simulink model "ModelArticulatingSpacecraftSolarPanelsforSunTrackingExample"  (R2025b)
settings: Solver=ode45  StartTime=0.0  StopTime=endTime  FixedStep=1/60  MaxStep=10  RelTol=1e-10  AbsTol=1e-10
undefined symbols (not defined in the file or in its folder): juliandate, panelY
libraries: aerolibutil x10, simulink x6, simulink_extras x6, aerolibsatdyn x4
settings Model: Creator=The MathWorks, Inc.  LastModifiedBy=Trent Jerome
settings OptimizationCC: ReuseModelBlockBuffer=off
settings ModelReferenceCC: EnableRefExpFcnMdlSchedulingChecks=on
settings RTWCC: GPUComputeCapability=3.5

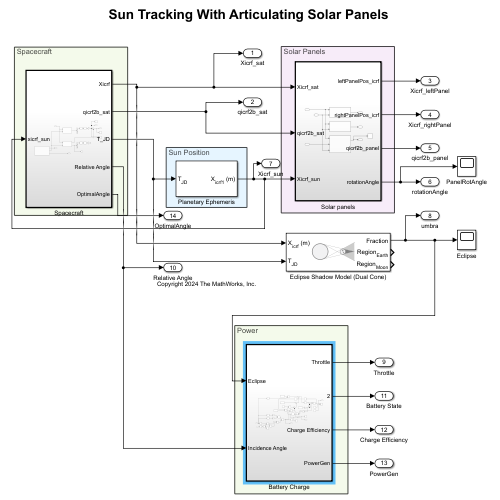
[thumbnail: Simulink's stored preview of the top-level diagram]
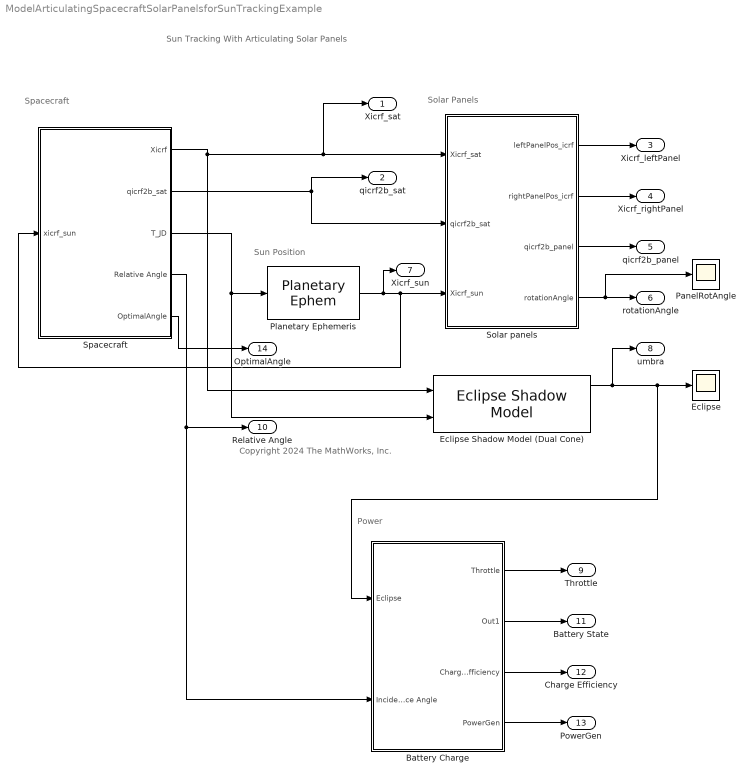
== system ModelArticulatingSpacecraftSolarPanelsforSunTrackingExample ==
  note: Sun Position
  note: Spacecraft
  note: Sun Tracking With Articulating Solar Panels
  note: Copyright 2024 The MathWorks, Inc.
  note: Solar Panels
  note: Power
  Battery Charge : Subsystem  TreatAsAtomicUnit=on
  Eclipse : Scope
      settings: ActiveDisplayYMinimum=-0.12499999999999997  ActiveDisplayYMaximum=1.125  DataLoggingVariableName=ScopeData2
  Eclipse Shadow Model (Dual Cone) : EclipseShadowModel  outputShadowRegion=on  timeSource=Port (Julian date)  useEphemerisDateRange=off  ephemerisEndDate=juliandate(2040, 1, 1)  action=Warning
  PanelRotAngle : Scope
      settings: ActiveDisplayYMinimum=0.6065745888777152  ActiveDisplayYMaximum=1.1603570435787431  DataLoggingVariableName=ScopeData12
  Planetary Ephemeris : PlanetaryEphem  units=m,m/s  target=Sun  outputVelocity=off
  Solar panels : Subsystem  TreatAsAtomicUnit=on
  Spacecraft : Subsystem  TreatAsAtomicUnit=on
  Xicrf_sat : Outport
  qicrf2b_sat : Outport  Port=2
  Xicrf_leftPanel : Outport  Port=3
  Xicrf_rightPanel : Outport  Port=4
  qicrf2b_panel : Outport  Port=5
  rotationAngle : Outport  Port=6
  Xicrf_sun : Outport  Port=7
  umbra : Outport  Port=8
  Throttle : Outport  Port=9
  Relative Angle : Outport  Port=10
  Battery State : Outport  Port=11
  Charge Efficiency : Outport  Port=12
  PowerGen : Outport  Port=13
  OptimalAngle : Outport  Port=14
  wires:
  Spacecraft/3(T_JD) -> Eclipse Shadow Model (Dual Cone)/2, Planetary Ephemeris/1
  Spacecraft/2(qicrf2b_sat) -> Solar panels/2(qicrf2b_sat), qicrf2b_sat/1
  Solar panels/2(rightPanelPos_icrf) -> Xicrf_rightPanel/1
  Solar panels/3(qicrf2b_panel) -> qicrf2b_panel/1
  Planetary Ephemeris/1 -> Xicrf_sun/1, Spacecraft/1(xicrf_sun), Solar panels/3(Xicrf_sun)
  Solar panels/1(leftPanelPos_icrf) -> Xicrf_leftPanel/1
  Solar panels/4(rotationAngle) -> PanelRotAngle/1, rotationAngle/1
  Spacecraft/1(Xicrf) -> Eclipse Shadow Model (Dual Cone)/1, Xicrf_sat/1, Solar panels/1(Xicrf_sat)
  Eclipse Shadow Model (Dual Cone)/1 -> umbra/1, Battery Charge/1(Eclipse), Eclipse/1
  Battery Charge/1(Throttle) -> Throttle/1
  Spacecraft/4(Relative Angle) -> Battery Charge/2(Incidence Angle), Relative Angle/1
  Battery Charge/2(Out1) -> Battery State/1
  Battery Charge/3(Charge Efficiency) -> Charge Efficiency/1
  Battery Charge/4(PowerGen) -> PowerGen/1
  Spacecraft/5(OptimalAngle) -> OptimalAngle/1

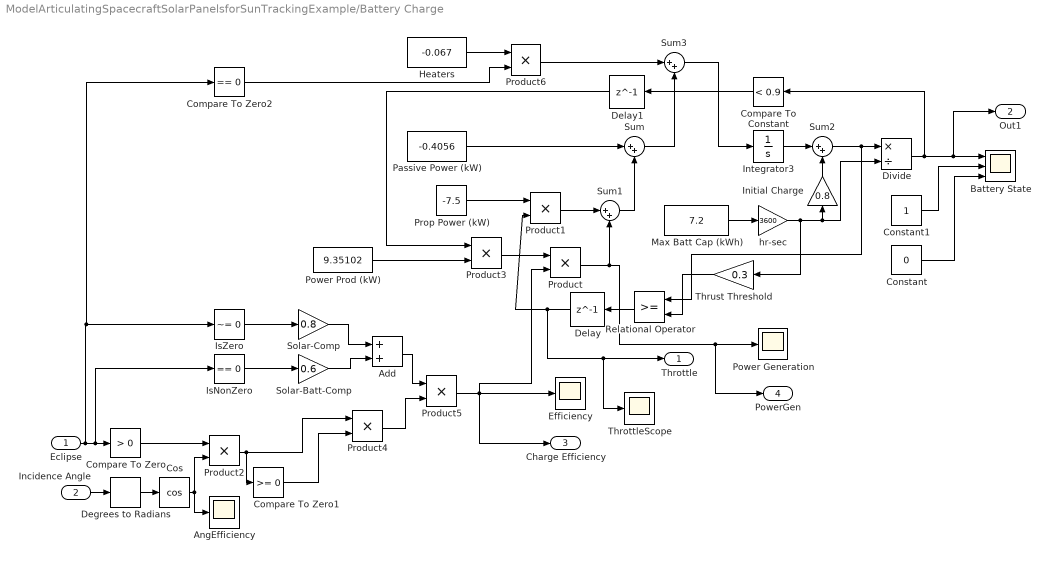
== system ModelArticulatingSpacecraftSolarPanelsforSunTrackingExample/Battery Charge ==
  Eclipse : Inport
  Incidence Angle : Inport  Port=2
  Add : Sum
  AngEfficiency : Scope
      settings: ActiveDisplayYMinimum=0.84489373386361877  ActiveDisplayYMaximum=1.0172340295545648  DataLoggingVariableName=ScopeData8
  Battery State : Scope  NumInputPorts=3
      settings: ActiveDisplayYMinimum=-0.12499999999999997  ActiveDisplayYMaximum=1.125  DataLoggingVariableName=ScopeData6
  Compare To Constant : simulink/Logic and Bit Operations/Compare To Constant  relop=<  const=0.9  OutDataTypeStr=boolean
  Compare To Zero : simulink/Logic and Bit Operations/Compare To Zero  relop=>  OutDataTypeStr=boolean
  Compare To Zero1 : simulink/Logic and Bit Operations/Compare To Zero  relop=>=  OutDataTypeStr=boolean
  Compare To Zero2 : simulink/Logic and Bit Operations/Compare To Zero  relop===  OutDataTypeStr=boolean
  Constant : Constant  Value=0
  Constant1 : Constant
  Cos : Trigonometry  Operator=cos
  Degrees to Radians : simulink_extras/Transformations/Degrees to Radians
  Delay : Delay  DelayLength=1  InitialCondition=0
  Delay1 : Delay  DelayLength=1  InitialCondition=0
  Divide : Product  Inputs=*/
  Efficiency : Scope
      settings: ActiveDisplayYMinimum=-0.1000000000042278  ActiveDisplayYMaximum=0.90000000003805047  DataLoggingVariableName=ScopeData9
  Heaters : Constant  Value=-0.067
  Initial Charge : Gain  Gain=0.8
  Integrator3 : Integrator
  IsNonZero : simulink/Logic and Bit Operations/Compare To Zero  relop===  OutDataTypeStr=boolean
      settings: LibrarySourceBlock=|
      | simulink/Quick Insert/Logic and Bit
      | Operations/IsNonZero
  IsZero : simulink/Logic and Bit Operations/Compare To Zero  relop=~=  OutDataTypeStr=boolean
      settings: LibrarySourceBlock=|
      | simulink/Quick Insert/Logic and Bit
      | Operations/IsZero
  Max Batt Cap (kWh) : Constant  Value=7.2
  Passive Power (kW) : Constant  Value=-0.4056
  Power Generation : Scope
      settings: ActiveDisplayYMinimum=-0.93510166556411412  ActiveDisplayYMaximum=8.41591499007703  DataLoggingVariableName=ScopeData13
  Power Prod (kW) : Constant  Value=9.35102
  Product{,1..6} (7 alike) : Product
  Prop Power (kW) : Constant  Value=-7.5
  Relational Operator : RelationalOperator  OutDataTypeStr=boolean  RndMeth=Simplest  InputSameDT=off
  Solar-Batt-Comp : Gain  Gain=0.6
  Solar-Comp : Gain  Gain=0.8
  Sum{,1..3} (4 alike) : Sum  Inputs=|++
  ThrottleScope : Scope
      settings: ActiveDisplayYMinimum=-0.12499999999999997  ActiveDisplayYMaximum=1.125  DataLoggingVariableName=ScopeData7
  Thrust Threshold : Gain  Gain=0.3
  hr-sec : Gain  Gain=3600
  Throttle : Outport
  Out1 : Outport  Port=2
  Charge Efficiency : Outport  Port=3
  PowerGen : Outport  Port=4
  wires:
  Eclipse/1 -> Compare To Zero2/1, IsZero/1, IsNonZero/1, Compare To Zero/1
  Passive Power (kW)/1 -> Sum/1
  Sum1/1 -> Sum/2
  Integrator3/1 -> Sum2/1
  Max Batt Cap (kWh)/1 -> hr-sec/1
  hr-sec/1 -> Divide/2, Initial Charge/1, Thrust Threshold/1
  Constant/1 -> Battery State/3
  Sum2/1 -> Divide/1, Relational Operator/1
  Initial Charge/1 -> Sum2/2
  Thrust Threshold/1 -> Relational Operator/2
  Relational Operator/1 -> Delay/1
  Prop Power (kW)/1 -> Product1/1
  Product1/1 -> Sum1/1
  Constant1/1 -> Battery State/2
  Divide/1 -> Compare To Constant/1, Out1/1, Battery State/1
  Compare To Zero/1 -> Product2/1
  Product2/1 -> Compare To Zero1/1, Product4/1
  Incidence Angle/1 -> Degrees to Radians/1
  Degrees to Radians/1 -> Cos/1
  Product3/1 -> Product/1
  Power Prod (kW)/1 -> Product3/2
  Compare To Constant/1 -> Delay1/1
  Delay/1 -> Product1/2, ThrottleScope/1, Throttle/1
  Delay1/1 -> Product3/1
  Compare To Zero1/1 -> Product4/2
  Cos/1 -> AngEfficiency/1, Product2/2
  Product4/1 -> Product5/2
  Product5/1 -> Product/2, Charge Efficiency/1, Efficiency/1
  Add/1 -> Product5/1
  Solar-Batt-Comp/1 -> Add/2
  Solar-Comp/1 -> Add/1
  IsZero/1 -> Solar-Comp/1
  IsNonZero/1 -> Solar-Batt-Comp/1
  Product/1 -> PowerGen/1, Power Generation/1, Sum1/2
  Sum3/1 -> Integrator3/1
  Sum/1 -> Sum3/2
  Heaters/1 -> Product6/1
  Product6/1 -> Sum3/1
  Compare To Zero2/1 -> Product6/2

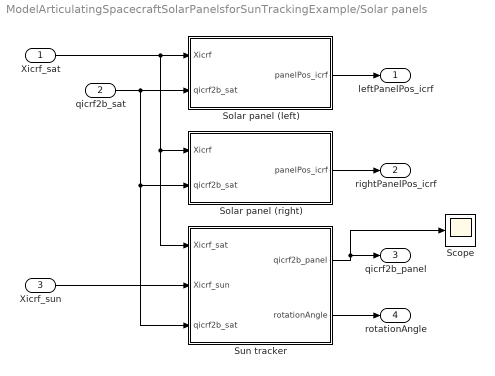
== system ModelArticulatingSpacecraftSolarPanelsforSunTrackingExample/Solar panels ==
  Xicrf_sat : Inport
  qicrf2b_sat : Inport  Port=2
  Xicrf_sun : Inport  Port=3
  Scope : Scope
      settings: ActiveDisplayYMinimum=-1  ActiveDisplayYMaximum=1
  Solar panel (left) : Subsystem
  Solar panel (right) : Subsystem
  Sun tracker : Subsystem
  leftPanelPos_icrf : Outport
  rightPanelPos_icrf : Outport  Port=2
  qicrf2b_panel : Outport  Port=3
  rotationAngle : Outport  Port=4
  wires:
  Sun tracker/1(qicrf2b_panel) -> Scope/1, qicrf2b_panel/1
  Solar panel (right)/1(panelPos_icrf) -> rightPanelPos_icrf/1
  qicrf2b_sat/1 -> Sun tracker/3(qicrf2b_sat), Solar panel (right)/2(qicrf2b_sat), Solar panel (left)/2(qicrf2b_sat)
  Xicrf_sat/1 -> Sun tracker/1(Xicrf_sat), Solar panel (right)/1(Xicrf), Solar panel (left)/1(Xicrf)
  Solar panel (left)/1(panelPos_icrf) -> leftPanelPos_icrf/1
  Sun tracker/2(rotationAngle) -> rotationAngle/1
  Xicrf_sun/1 -> Sun tracker/2(Xicrf_sun)

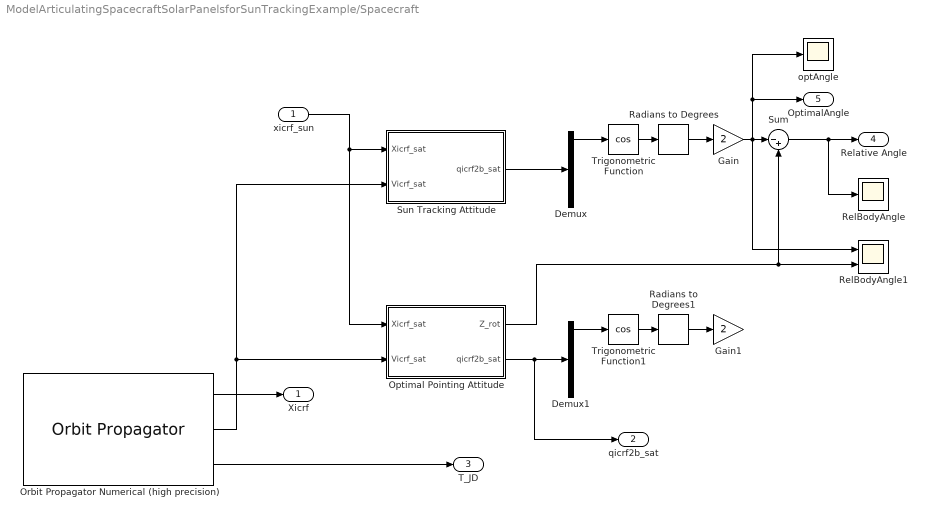
== system ModelArticulatingSpacecraftSolarPanelsforSunTrackingExample/Spacecraft ==
  xicrf_sun : Inport
  Demux : Demux
  Demux1 : Demux
  Gain : Gain  Gain=2
  Gain1 : Gain  Gain=2
  Optimal Pointing Attitude : Subsystem  TreatAsAtomicUnit=on
  Orbit Propagator Numerical (high precision) : OrbitPropagator  propagator=Numerical (high precision)  startDate=initialTimeJD  semiMajorAxis=semiMajorAxis  eccentricity=eccentricity  inclination=inclination  raan=rightAscensionOfAscendingNode  argPeriapsis=argumentOfPeriapsis  trueAnomaly=trueAnomaly  inertialPosition=[3649700.0 3308200.0 -4676600.0]  inertialVelocity=[-2750.8 6666.4 2573.4]  fixedPosition=[-4142689.0 -2676864.7 -4669861.6]  fixedVelocity=[1452.7 -6720.7 2568.1]  gravityModel=Oblate ellipsoid (J2)  customR=3396200  customMu=4.305e13  customJ2=1.0826269e-03  customOmega=4.06125949e-3  useEOPs=off
  Radians to Degrees : simulink_extras/Transformations/Radians to Degrees
  Radians to Degrees1 : simulink_extras/Transformations/Radians to Degrees
  RelBodyAngle : Scope
      settings: ActiveDisplayYMinimum=-7.94352171426871  ActiveDisplayYMaximum=32.32470810282144  DataLoggingVariableName=ScopeData5
  RelBodyAngle1 : Scope  NumInputPorts=2
      settings: ActiveDisplayYMinimum=55.616290533406783  ActiveDisplayYMaximum=121.14436663647109  DataLoggingVariableName=ScopeData4
  Sum : Sum  Inputs=|-+
  "Sun Tracking Attitude " : Subsystem  TreatAsAtomicUnit=on
  Trigonometric Function : Trigonometry  Operator=cos
  Trigonometric Function1 : Trigonometry  Operator=cos
  optAngle : Scope
      settings: ActiveDisplayYMinimum=-1  ActiveDisplayYMaximum=1  DataLoggingVariableName=ScopeData10
  Xicrf : Outport
  qicrf2b_sat : Outport  Port=2
  T_JD : Outport  Port=3
  Relative Angle : Outport  Port=4
  OptimalAngle : Outport  Port=5
  wires:
  Orbit Propagator Numerical (high precision)/3 -> T_JD/1
  Orbit Propagator Numerical (high precision)/1 -> Xicrf/1
  Orbit Propagator Numerical (high precision)/2 -> Optimal Pointing Attitude/2(Vicrf_sat), "Sun Tracking Attitude "/2(Vicrf_sat)
  Demux/1 -> Trigonometric Function/1
  Trigonometric Function/1 -> Radians to Degrees/1
  Gain/1 -> RelBodyAngle1/1, OptimalAngle/1, optAngle/1, Sum/1
  Radians to Degrees/1 -> Gain/1
  "Sun Tracking Attitude "/1(qicrf2b_sat) -> Demux/1
  Sum/1 -> RelBodyAngle/1, Relative Angle/1
  xicrf_sun/1 -> Optimal Pointing Attitude/1(Xicrf_sat), "Sun Tracking Attitude "/1(Xicrf_sat)
  Trigonometric Function1/1 -> Radians to Degrees1/1
  Demux1/1 -> Trigonometric Function1/1
  Radians to Degrees1/1 -> Gain1/1
  Optimal Pointing Attitude/2(qicrf2b_sat) -> qicrf2b_sat/1, Demux1/1
  Optimal Pointing Attitude/1(Z_rot) -> Sum/2, RelBodyAngle1/2

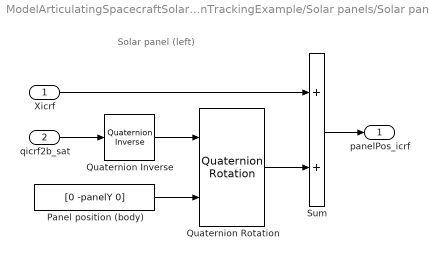
== system ModelArticulatingSpacecraftSolarPanelsforSunTrackingExample/Solar panels/Solar panel (left) ==
  note: Solar panel (left)
  Xicrf : Inport
  qicrf2b_sat : Inport  Port=2
  Panel position (body) : Constant  Value=[0 -panelY 0]
  Quaternion Inverse : aerolibutil/Quaternion Inverse
  Quaternion Rotation : aerolibutil/Quaternion Rotation
  Sum : Sum
  panelPos_icrf : Outport
  wires:
  Quaternion Inverse/1 -> Quaternion Rotation/1
  Quaternion Rotation/1 -> Sum/2
  qicrf2b_sat/1 -> Quaternion Inverse/1
  Panel position (body)/1 -> Quaternion Rotation/2
  Xicrf/1 -> Sum/1
  Sum/1 -> panelPos_icrf/1

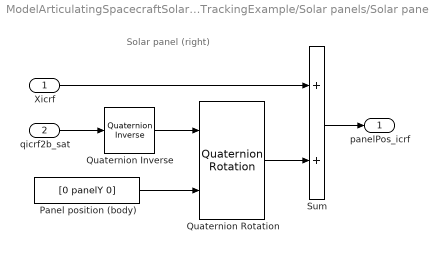
== system ModelArticulatingSpacecraftSolarPanelsforSunTrackingExample/Solar panels/Solar panel (right) ==
  note: Solar panel (right)
  Xicrf : Inport
  qicrf2b_sat : Inport  Port=2
  Panel position (body) : Constant  Value=[0 panelY 0]
  Quaternion Inverse : aerolibutil/Quaternion Inverse
  Quaternion Rotation : aerolibutil/Quaternion Rotation
  Sum : Sum
  panelPos_icrf : Outport
  wires:
  Quaternion Inverse/1 -> Quaternion Rotation/1
  Quaternion Rotation/1 -> Sum/2
  qicrf2b_sat/1 -> Quaternion Inverse/1
  Panel position (body)/1 -> Quaternion Rotation/2
  Xicrf/1 -> Sum/1
  Sum/1 -> panelPos_icrf/1

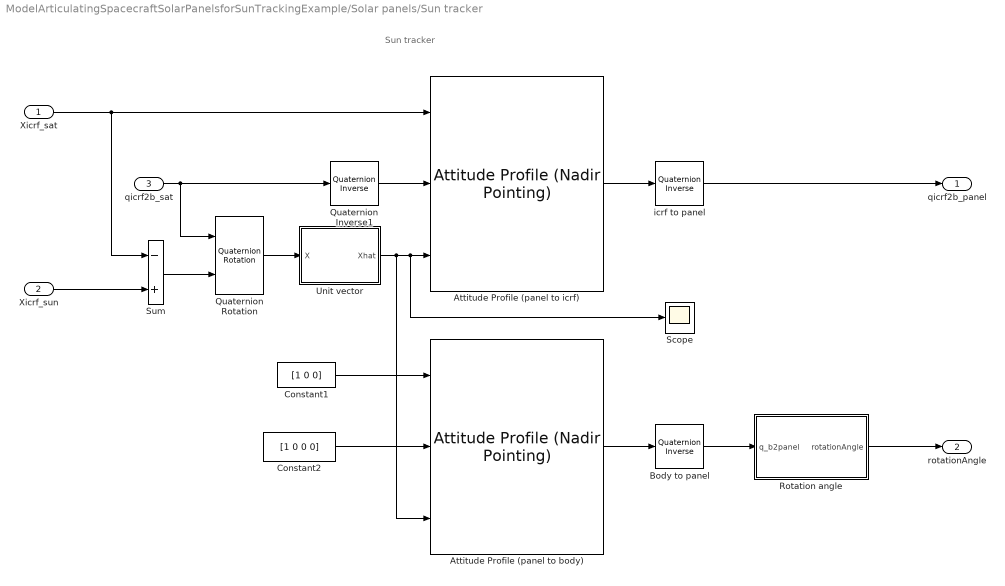
== system ModelArticulatingSpacecraftSolarPanelsforSunTrackingExample/Solar panels/Sun tracker ==
  note: Sun tracker
  Xicrf_sat : Inport
  Xicrf_sun : Inport  Port=2
  qicrf2b_sat : Inport  Port=3
  Attitude Profile (panel to body) : aerolibsatdyn/Attitude Profile (Nadir Pointing)  outputError=off  outputFinalAttitude=on  portFrame=ICRF  pointingMode=Custom  celestialTarget=Sun  tunablePointing=off  primaryAlignmentSrc=Dialog  primaryAlignment=[0 1 0]  secondaryAlignmentSrc=Dialog  secondaryAlignment=[0 0 1]  constraintFrame=Body-frame  primaryConstraintSrc=Dialog  primaryConstraint=[0 1 0]  secondaryConstraintSrc=Port  secondaryConstraint=[0 1 0]
  Attitude Profile (panel to icrf) : aerolibsatdyn/Attitude Profile (Nadir Pointing)  outputError=off  outputFinalAttitude=on  portFrame=ICRF  pointingMode=Custom  celestialTarget=Sun  tunablePointing=off  primaryAlignmentSrc=Dialog  primaryAlignment=[0 1 0]  secondaryAlignmentSrc=Dialog  secondaryAlignment=[0 0 1]  constraintFrame=Body-frame  primaryConstraintSrc=Dialog  primaryConstraint=[0 1 0]  secondaryConstraintSrc=Port  secondaryConstraint=[0 1 0]
  Body to panel : aerolibutil/Quaternion Inverse
  Constant1 : Constant  Value=[1 0 0]
  Constant2 : Constant  Value=[1 0 0 0]
  Quaternion Inverse1 : aerolibutil/Quaternion Inverse
  Quaternion Rotation : aerolibutil/Quaternion Rotation
  Rotation angle : Subsystem
  Scope : Scope
      settings: ActiveDisplayYMinimum=-1  ActiveDisplayYMaximum=1  DataLoggingVariableName=ScopeData3
  Sum : Sum  Inputs=-+
  Unit vector : Subsystem
  icrf to panel : aerolibutil/Quaternion Inverse
  qicrf2b_panel : Outport
  rotationAngle : Outport  Port=2
  wires:
  icrf to panel/1 -> qicrf2b_panel/1
  qicrf2b_sat/1 -> Quaternion Rotation/1, Quaternion Inverse1/1
  Quaternion Inverse1/1 -> Attitude Profile (panel to icrf)/2
  Xicrf_sat/1 -> Sum/1, Attitude Profile (panel to icrf)/1
  Attitude Profile (panel to icrf)/1 -> icrf to panel/1
  Quaternion Rotation/1 -> Unit vector/1(X)
  Attitude Profile (panel to body)/1 -> Body to panel/1
  Constant1/1 -> Attitude Profile (panel to body)/1
  Constant2/1 -> Attitude Profile (panel to body)/2
  Body to panel/1 -> Rotation angle/1(q_b2panel)
  Rotation angle/1(rotationAngle) -> rotationAngle/1
  Xicrf_sun/1 -> Sum/2
  Sum/1 -> Quaternion Rotation/2
  Unit vector/1(Xhat) -> Scope/1, Attitude Profile (panel to icrf)/3, Attitude Profile (panel to body)/3

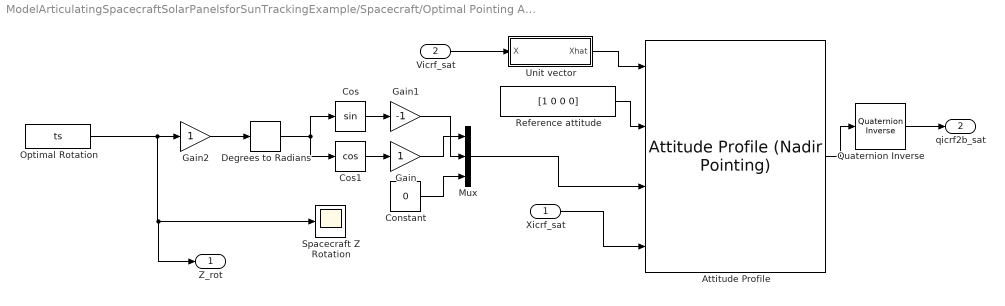
== system ModelArticulatingSpacecraftSolarPanelsforSunTrackingExample/Spacecraft/Optimal Pointing Attitude ==
  Xicrf_sat : Inport
  Vicrf_sat : Inport  Port=2
  Attitude Profile : aerolibsatdyn/Attitude Profile (Nadir Pointing)  outputError=off  outputFinalAttitude=on  portFrame=ICRF  pointingMode=Point at nadir  celestialTarget=Sun  tunablePointing=off  primaryAlignmentSrc=Dialog  primaryAlignment=[0 0 1]  secondaryAlignmentSrc=Port  secondaryAlignment=[0 1 0]  constraintFrame=ICRF  primaryConstraintSrc=Port  primaryConstraint=[1 0 0]  secondaryConstraintSrc=Port  secondaryConstraint=[0 0 1]
  Constant : Constant  Value=0
  Cos : Trigonometry
  Cos1 : Trigonometry  Operator=cos
  Degrees to Radians : simulink_extras/Transformations/Degrees to Radians
  Gain : Gain
  Gain1 : Gain  Gain=-1
  Gain2 : Gain
  Mux : Mux  Inputs=3
  Optimal Rotation : FromWorkspace  VariableName=ts  SampleTime=-1
  Quaternion Inverse : aerolibutil/Quaternion Inverse
  Reference attitude : Constant  Value=[1 0 0 0]
  Spacecraft Z Rotation : Scope
      settings: ActiveDisplayYMinimum=110.6463369139733  ActiveDisplayYMaximum=110.68306278370297  DataLoggingVariableName=ScopeData11
  Unit vector : Subsystem
  Z_rot : Outport
  qicrf2b_sat : Outport  Port=2
  wires:
  Quaternion Inverse/1 -> qicrf2b_sat/1
  Vicrf_sat/1 -> Unit vector/1(X)
  Attitude Profile/1 -> Quaternion Inverse/1
  Reference attitude/1 -> Attitude Profile/2
  Unit vector/1(Xhat) -> Attitude Profile/1
  Xicrf_sat/1 -> Attitude Profile/4
  Cos/1 -> Gain1/1
  Cos1/1 -> Gain/1
  Optimal Rotation/1 -> Z_rot/1, Spacecraft Z Rotation/1, Gain2/1
  Degrees to Radians/1 -> Cos1/1, Cos/1
  Gain2/1 -> Degrees to Radians/1
  Mux/1 -> Attitude Profile/3
  Constant/1 -> Mux/3
  Gain/1 -> Mux/1
  Gain1/1 -> Mux/2

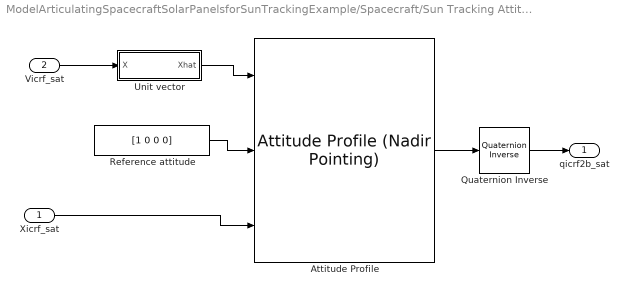
== system ModelArticulatingSpacecraftSolarPanelsforSunTrackingExample/Spacecraft/Sun Tracking Attitude  ==
  Xicrf_sat : Inport
  Vicrf_sat : Inport  Port=2
  Attitude Profile : aerolibsatdyn/Attitude Profile (Nadir Pointing)  outputError=off  outputFinalAttitude=on  portFrame=ICRF  pointingMode=Point at nadir  celestialTarget=Sun  tunablePointing=off  primaryAlignmentSrc=Dialog  primaryAlignment=[0 0 1]  secondaryAlignmentSrc=Dialog  secondaryAlignment=[1 0 0]  constraintFrame=ICRF  primaryConstraintSrc=Port  primaryConstraint=[1 0 0]  secondaryConstraintSrc=Port  secondaryConstraint=[0 0 1]
  Quaternion Inverse : aerolibutil/Quaternion Inverse
  Reference attitude : Constant  Value=[1 0 0 0]
  Unit vector : Subsystem
  qicrf2b_sat : Outport
  wires:
  Quaternion Inverse/1 -> qicrf2b_sat/1
  Vicrf_sat/1 -> Unit vector/1(X)
  Attitude Profile/1 -> Quaternion Inverse/1
  Reference attitude/1 -> Attitude Profile/2
  Unit vector/1(Xhat) -> Attitude Profile/1
  Xicrf_sat/1 -> Attitude Profile/3

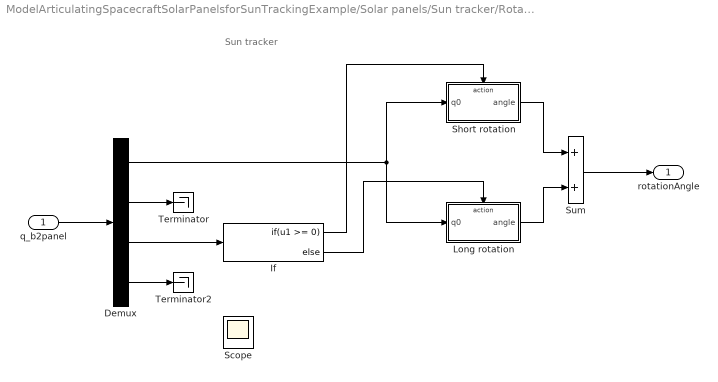
== system ModelArticulatingSpacecraftSolarPanelsforSunTrackingExample/Solar panels/Sun tracker/Rotation angle ==
  note: Sun tracker
  q_b2panel : Inport
  Demux : Demux
  If : If  IfExpression=u1 >= 0
  Long rotation : Subsystem  TreatAsAtomicUnit=on
  Scope : Scope
      settings: ActiveDisplayYMinimum=-1  ActiveDisplayYMaximum=1
  Short rotation : Subsystem  TreatAsAtomicUnit=on
  Sum : Sum
  Terminator : Terminator
  Terminator2 : Terminator
  rotationAngle : Outport
  wires:
  Long rotation/1(angle) -> Sum/2
  Short rotation/1(angle) -> Sum/1
  Demux/1 -> Short rotation/1(q0), Long rotation/1(q0)
  Demux/3 -> If/1
  If/2 -> Long rotation/Action
  If/1 -> Short rotation/Action
  Sum/1 -> rotationAngle/1
  q_b2panel/1 -> Demux/1
  Demux/2 -> Terminator/1
  Demux/4 -> Terminator2/1

== system ModelArticulatingSpacecraftSolarPanelsforSunTrackingExample/Solar panels/Sun tracker/Unit vector ==
  X : Inport
  Divide : Product  Inputs=*/
  Dot Product : DotProduct  OutDataTypeStr=Inherit: Inherit via internal rule
  Sqrt : Sqrt
  Xhat : Outport
  wires:
  Dot Product/1 -> Sqrt/1
  X/1 -> Divide/1, Dot Product/2, Dot Product/1
  Divide/1 -> Xhat/1
  Sqrt/1 -> Divide/2

== system ModelArticulatingSpacecraftSolarPanelsforSunTrackingExample/Spacecraft/Optimal Pointing Attitude/Unit vector ==
  X : Inport
  Divide : Product  Inputs=*/
  Dot Product : DotProduct  OutDataTypeStr=Inherit: Inherit via internal rule
  Xhat : Outport
  wires:
  Dot Product/1 -> Divide/2
  X/1 -> Divide/1, Dot Product/2, Dot Product/1
  Divide/1 -> Xhat/1

== system ModelArticulatingSpacecraftSolarPanelsforSunTrackingExample/Spacecraft/Sun Tracking Attitude /Unit vector ==
  X : Inport
  Divide : Product  Inputs=*/
  Dot Product : DotProduct  OutDataTypeStr=Inherit: Inherit via internal rule
  Xhat : Outport
  wires:
  Dot Product/1 -> Divide/2
  X/1 -> Divide/1, Dot Product/2, Dot Product/1
  Divide/1 -> Xhat/1

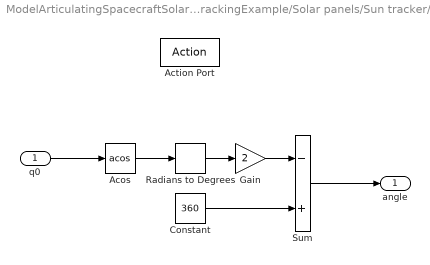
== system ModelArticulatingSpacecraftSolarPanelsforSunTrackingExample/Solar panels/Sun tracker/Rotation angle/Long rotation ==
  q0 : Inport
  Action Port : ActionPort  ActionPortLabel=else
  Acos : Trigonometry  Operator=acos
  Constant : Constant  Value=360
  Gain : Gain  Gain=2
  Radians to Degrees : simulink_extras/Transformations/Radians to Degrees
  Sum : Sum  Inputs=-+
  angle : Outport  OutputWhenDisabled=reset  InitialOutput=0
  wires:
  Acos/1 -> Radians to Degrees/1
  q0/1 -> Acos/1
  Radians to Degrees/1 -> Gain/1
  Constant/1 -> Sum/2
  Sum/1 -> angle/1
  Gain/1 -> Sum/1

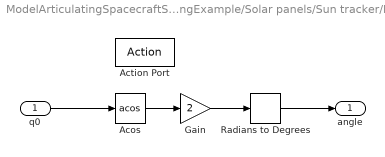
== system ModelArticulatingSpacecraftSolarPanelsforSunTrackingExample/Solar panels/Sun tracker/Rotation angle/Short rotation ==
  q0 : Inport
  Action Port : ActionPort  ActionPortLabel=if(u1 >= 0)
  Acos : Trigonometry  Operator=acos
  Gain : Gain  Gain=2
  Radians to Degrees : simulink_extras/Transformations/Radians to Degrees
  angle : Outport  OutputWhenDisabled=reset  InitialOutput=0
  wires:
  q0/1 -> Acos/1
  Acos/1 -> Gain/1
  Radians to Degrees/1 -> angle/1
  Gain/1 -> Radians to Degrees/1
